simulink model "mrefrobotarm_modified_previous_y_previous_u_previous_ref"  (R2018b)
settings: Solver=FixedStepAuto  StartTime=0.0  StopTime=10  RelTol=1e-3  AbsTol=1e-6
undefined symbols (not defined in the file or in its folder): options, sfunxy2
libraries: neural x949, simulink x1
(part 7 of 31)

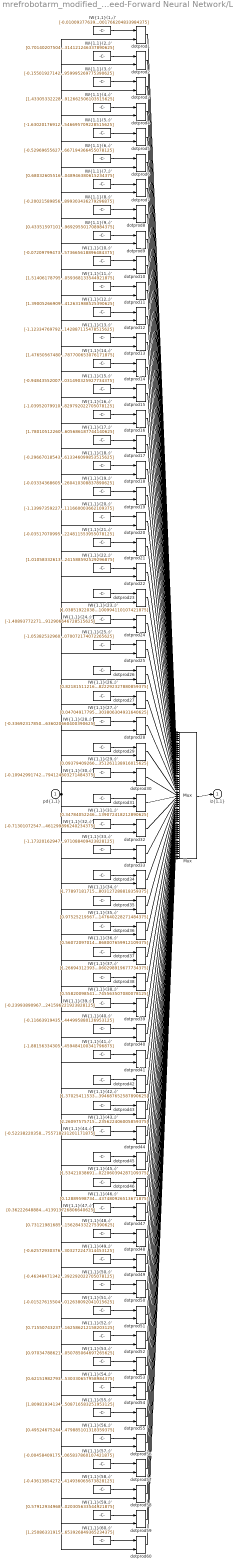
== system mrefrobotarm_modified_previous_y_previous_u_previous_ref/Feed-Forward Neural Network/Layer 1/IW{1,1} ==
  "pd{1,1}" : Inport  PortDimensions=8
      mask Display: e = 0.06;c1 = [120 230 180]/255;c2 = ([120 230 180]+0)/(256+128);c3 = ([120 230 180]+128)/(256+128);patch([0 1 1 0],[0 0 1 1],c1);patch([0 1 1 1-e 1-e 0+e],[0 0 1 1-e 0+e 0+e],c2);patch([0 0 1 1-e 0+e 0+e],[0 1 1 1-e 1-e 0+e],c3);plot([0 1 1 0 0],[0 0 1 1 0]);
  "IW{1,1}(1,:)'" : Constant  Value=[-0.01009377639347205403430596248881556675769388675689697265625;-0.81917856322471305219323767232708632946014404296875;-1.0919884952677578748847508904873393476009368896484375;-0.3232934690770914443191941245459020137786865234375;1.0371983069879358030362936915480531752109527587890625;0.332566501638959455267041676052031107246875762939453125;-0.72214891052584950781323414048529230058193206787109375;0.41554839927694986467798798912554048001766204833984375]
      mask Display: e = 0.06;c1 = [120 150 230]/255;c2 = ([120 150 230]+0)/383;c3 = ([120 150 230]+128)/383;patch([0 1 1 0],[0 0 1 1],c1);patch([0 1 1 1-e 1-e 0+e],[0 0 1 1-e 0+e 0+e],c2);patch([0 0 1 1-e 0+e 0+e],[0 1 1 1-e 1-e 0+e],c3);plot([0 1 1 0 0],[0 0 1 1 0]);disp('Weights');
  "IW{1,1}(10,:)'" : Constant  Value=[-0.0720979947310176616515065006751683540642261505126953125;1.1315755262161395489073356657172553241252899169921875;-0.69309946443650216618692638803622685372829437255859375;-0.1580631105350375487095249127378338016569614410400390625;-0.70708492198913841519924972089938819408416748046875;-0.9763414859311836391242422905634157359600067138671875;0.56334312317556867188983460437157191336154937744140625;-0.319187622528195491522495785829960368573665618896484375]
      mask Display: e = 0.06;c1 = [120 150 230]/255;c2 = ([120 150 230]+0)/383;c3 = ([120 150 230]+128)/383;patch([0 1 1 0],[0 0 1 1],c1);patch([0 1 1 1-e 1-e 0+e],[0 0 1 1-e 0+e 0+e],c2);patch([0 0 1 1-e 0+e 0+e],[0 1 1 1-e 1-e 0+e],c3);plot([0 1 1 0 0],[0 0 1 1 0]);disp('Weights');
  "IW{1,1}(11,:)'" : Constant  Value=[1.514061787956713533986885522608645260334014892578125;-0.41268670620541703097927666021860204637050628662109375;-0.133355521691774558945553508237935602664947509765625;1.4642596982166242725043048267252743244171142578125;-0.92497175926368180309822264462127350270748138427734375;-0.0687966183859873847694643700378946959972381591796875;0.715766413497218589867543414584361016750335693359375;0.2974930277251821575390522411908023059368133544921875]
      mask Display: e = 0.06;c1 = [120 150 230]/255;c2 = ([120 150 230]+0)/383;c3 = ([120 150 230]+128)/383;patch([0 1 1 0],[0 0 1 1],c1);patch([0 1 1 1-e 1-e 0+e],[0 0 1 1-e 0+e 0+e],c2);patch([0 0 1 1-e 0+e 0+e],[0 1 1 1-e 1-e 0+e],c3);plot([0 1 1 0 0],[0 0 1 1 0]);disp('Weights');
  "IW{1,1}(12,:)'" : Constant  Value=[1.390052669090437120757997035980224609375;0.002873883030498494174642676313169431523419916629791259765625;-0.265197877421132155451033440840546973049640655517578125;-0.2012360557710944630738225669119856320321559906005859375;-0.73320460680185417512433332376531325280666351318359375;-0.0226500905621143909518533376967752701602876186370849609375;-0.057008062463787374796186924186258693225681781768798828125;-0.9276377305383221028023399412631988525390625]
      mask Display: e = 0.06;c1 = [120 150 230]/255;c2 = ([120 150 230]+0)/383;c3 = ([120 150 230]+128)/383;patch([0 1 1 0],[0 0 1 1],c1);patch([0 1 1 1-e 1-e 0+e],[0 0 1 1-e 0+e 0+e],c2);patch([0 0 1 1-e 0+e 0+e],[0 1 1 1-e 1-e 0+e],c3);plot([0 1 1 0 0],[0 0 1 1 0]);disp('Weights');
  "IW{1,1}(13,:)'" : Constant  Value=[-1.1233476979256022953990168389282189309597015380859375;-1.2393693114673052235730210668407380580902099609375;0.7914246902064994149128551725880242884159088134765625;-0.274134462483511198716001899811089970171451568603515625;-0.7315570973101059859544648134033195674419403076171875;0.428567667581298328283168075358844362199306488037109375;1.018170137932393526369878600235097110271453857421875;0.49897495766321908750029479051590897142887115478515625]
      mask Display: e = 0.06;c1 = [120 150 230]/255;c2 = ([120 150 230]+0)/383;c3 = ([120 150 230]+128)/383;patch([0 1 1 0],[0 0 1 1],c1);patch([0 1 1 1-e 1-e 0+e],[0 0 1 1-e 0+e 0+e],c2);patch([0 0 1 1-e 0+e 0+e],[0 1 1 1-e 1-e 0+e],c3);plot([0 1 1 0 0],[0 0 1 1 0]);disp('Weights');
  "IW{1,1}(14,:)'" : Constant  Value=[1.4765056748086795579411045764572918415069580078125;-0.90659967261472174104852683740318752825260162353515625;1.1508044721540480193056055213673971593379974365234375;-1.0136176640992273778607568601728416979312896728515625;-0.07767755483619455392219066425241180695593357086181640625;0.57299887905671254006989556728512980043888092041015625;0.449131233253424244633578155116993002593517303466796875;0.1613292379590309522097157923781196586787700653076171875]
      mask Display: e = 0.06;c1 = [120 150 230]/255;c2 = ([120 150 230]+0)/383;c3 = ([120 150 230]+128)/383;patch([0 1 1 0],[0 0 1 1],c1);patch([0 1 1 1-e 1-e 0+e],[0 0 1 1-e 0+e 0+e],c2);patch([0 0 1 1-e 0+e 0+e],[0 1 1 1-e 1-e 0+e],c3);plot([0 1 1 0 0],[0 0 1 1 0]);disp('Weights');
  "IW{1,1}(15,:)'" : Constant  Value=[-0.94843552007180209617587252068915404379367828369140625;-0.455396495188023886502293180456035770475864410400390625;-0.71794256963177804919951086048968136310577392578125;-0.259356227336552891404863885327358730137348175048828125;-0.6977913420825629930988043270190246403217315673828125;1.4367856825259675002115500319632701575756072998046875;0.38097748667274744516220152945606969296932220458984375;-1.2386509874698869992926120175980031490325927734375]
      mask Display: e = 0.06;c1 = [120 150 230]/255;c2 = ([120 150 230]+0)/383;c3 = ([120 150 230]+128)/383;patch([0 1 1 0],[0 0 1 1],c1);patch([0 1 1 1-e 1-e 0+e],[0 0 1 1-e 0+e 0+e],c2);patch([0 0 1 1-e 0+e 0+e],[0 1 1 1-e 1-e 0+e],c3);plot([0 1 1 0 0],[0 0 1 1 0]);disp('Weights');
  "IW{1,1}(16,:)'" : Constant  Value=[-1.03952079910626782321969585609622299671173095703125;0.274781364075693590454108061749138869345188140869140625;-1.0171273753363585523601386739755980670452117919921875;-0.03878824548100874569644958000935730524361133575439453125;0.193393524233432978487456921357079409062862396240234375;0.832640986442755082208577732671983540058135986328125;-0.7503621573611758410748961978242732584476470947265625;-1.01693222204544486686472737346775829792022705078125]
      mask Display: e = 0.06;c1 = [120 150 230]/255;c2 = ([120 150 230]+0)/383;c3 = ([120 150 230]+128)/383;patch([0 1 1 0],[0 0 1 1],c1);patch([0 1 1 1-e 1-e 0+e],[0 0 1 1-e 0+e 0+e],c2);patch([0 0 1 1-e 0+e 0+e],[0 1 1 1-e 1-e 0+e],c3);plot([0 1 1 0 0],[0 0 1 1 0]);disp('Weights');
  "IW{1,1}(17,:)'" : Constant  Value=[1.7801051226057931220481123091303743422031402587890625;1.3780535999959975246298427009605802595615386962890625;0.1885363073008298473443034026786335743963718414306640625;0.365832667926227206312006501320865936577320098876953125;0.6397823368767736607054530395544134080410003662109375;0.379418365358508646867363722776644863188266754150390625;-0.26533033038375464229829958640038967132568359375;0.30752361343576029018009876381256617605686187744140625]
      mask Display: e = 0.06;c1 = [120 150 230]/255;c2 = ([120 150 230]+0)/383;c3 = ([120 150 230]+128)/383;patch([0 1 1 0],[0 0 1 1],c1);patch([0 1 1 1-e 1-e 0+e],[0 0 1 1-e 0+e 0+e],c2);patch([0 0 1 1-e 0+e 0+e],[0 1 1 1-e 1-e 0+e],c3);plot([0 1 1 0 0],[0 0 1 1 0]);disp('Weights');
  "IW{1,1}(18,:)'" : Constant  Value=[-0.296670185432604427422376147660543210804462432861328125;-0.376072809350395387273380265469313599169254302978515625;-0.742727493493180901396044646389782428741455078125;0.86593116784423240783752362403902225196361541748046875;1.37064929615764707904190800036303699016571044921875;-0.59077170502804399188079287341679446399211883544921875;-0.150853642388064368429212436240050010383129119873046875;-0.81451885680998670213881496238172985613346099853515625]
      mask Display: e = 0.06;c1 = [120 150 230]/255;c2 = ([120 150 230]+0)/383;c3 = ([120 150 230]+128)/383;patch([0 1 1 0],[0 0 1 1],c1);patch([0 1 1 1-e 1-e 0+e],[0 0 1 1-e 0+e 0+e],c2);patch([0 0 1 1-e 0+e 0+e],[0 1 1 1-e 1-e 0+e],c3);plot([0 1 1 0 0],[0 0 1 1 0]);disp('Weights');
  "IW{1,1}(19,:)'" : Constant  Value=[-0.033343686056520986660256511413535918109118938446044921875;-0.5300304829595254840768348003621213138103485107421875;-0.66380007316216460555580169966560788452625274658203125;1.4047136071211827612614797544665634632110595703125;-1.4498046029545166302199277197360061109066009521484375;0.60291678893256517302035035754670388996601104736328125;-0.08866355731311535703920156947788200341165065765380859375;-0.3794826026320132772440274493419565260410308837890625]
      mask Display: e = 0.06;c1 = [120 150 230]/255;c2 = ([120 150 230]+0)/383;c3 = ([120 150 230]+128)/383;patch([0 1 1 0],[0 0 1 1],c1);patch([0 1 1 1-e 1-e 0+e],[0 0 1 1-e 0+e 0+e],c2);patch([0 0 1 1-e 0+e 0+e],[0 1 1 1-e 1-e 0+e],c3);plot([0 1 1 0 0],[0 0 1 1 0]);disp('Weights');
  "IW{1,1}(2,:)'" : Constant  Value=[0.70140207504615859068763938921620137989521026611328125;0.50190548995443251545367502330918796360492706298828125;1.178018179952304844704258357523940503597259521484375;1.2397835887663470888497840860509313642978668212890625;1.2796434023332323715038683076272718608379364013671875;-0.91185964599935942498376562070916406810283660888671875;-0.53150803539821700471890153494314290583133697509765625;0.60564464089634706400744335041963495314121246337890625]
      mask Display: e = 0.06;c1 = [120 150 230]/255;c2 = ([120 150 230]+0)/383;c3 = ([120 150 230]+128)/383;patch([0 1 1 0],[0 0 1 1],c1);patch([0 1 1 1-e 1-e 0+e],[0 0 1 1-e 0+e 0+e],c2);patch([0 0 1 1-e 0+e 0+e],[0 1 1 1-e 1-e 0+e],c3);plot([0 1 1 0 0],[0 0 1 1 0]);disp('Weights');
  "IW{1,1}(20,:)'" : Constant  Value=[-1.139973592271053437485761605785228312015533447265625;0.922414963173714408384284979547373950481414794921875;0.573062580631909401773782519740052521228790283203125;-1.0638984585657997872232272129622288048267364501953125;0.26000003990170894585531868870020844042301177978515625;-1.0082968466580883859506911903736181557178497314453125;-0.427975846736409037962545198752195574343204498291015625;-0.404524086197522725338870941413915716111660003662109375]
      mask Display: e = 0.06;c1 = [120 150 230]/255;c2 = ([120 150 230]+0)/383;c3 = ([120 150 230]+128)/383;patch([0 1 1 0],[0 0 1 1],c1);patch([0 1 1 1-e 1-e 0+e],[0 0 1 1-e 0+e 0+e],c2);patch([0 0 1 1-e 0+e 0+e],[0 1 1 1-e 1-e 0+e],c3);plot([0 1 1 0 0],[0 0 1 1 0]);disp('Weights');
  "IW{1,1}(21,:)'" : Constant  Value=[-0.035170709953433833272473663100754492916166782379150390625;-0.2048825226713566205472005776755395345389842987060546875;1.02054460527438362049679199117235839366912841796875;-1.0483393952073327692886550721595995128154754638671875;0.218116613354659649726130510316579602658748626708984375;-1.2810290950311611357648189368774183094501495361328125;0.9860421910966181702207222770084626972675323486328125;-0.30606358720429505115845358886872418224811553955078125]
      mask Display: e = 0.06;c1 = [120 150 230]/255;c2 = ([120 150 230]+0)/383;c3 = ([120 150 230]+128)/383;patch([0 1 1 0],[0 0 1 1],c1);patch([0 1 1 1-e 1-e 0+e],[0 0 1 1-e 0+e 0+e],c2);patch([0 0 1 1-e 0+e 0+e],[0 1 1 1-e 1-e 0+e],c3);plot([0 1 1 0 0],[0 0 1 1 0]);disp('Weights');
  "IW{1,1}(22,:)'" : Constant  Value=[1.010583326137901583052780551952309906482696533203125;-0.34255096084721647908821751116192899644374847412109375;0.49744289643764882935528248708578757941722869873046875;0.81639407608297276386366547740180976688861846923828125;0.268321118702407546141586180965532548725605010986328125;-1.0453340103508159675271826927200891077518463134765625;1.0355195133497721027282523209578357636928558349609375;-0.53749069554478612342762744447099976241588592529296875]
      mask Display: e = 0.06;c1 = [120 150 230]/255;c2 = ([120 150 230]+0)/383;c3 = ([120 150 230]+128)/383;patch([0 1 1 0],[0 0 1 1],c1);patch([0 1 1 1-e 1-e 0+e],[0 0 1 1-e 0+e 0+e],c2);patch([0 0 1 1-e 0+e 0+e],[0 1 1 1-e 1-e 0+e],c3);plot([0 1 1 0 0],[0 0 1 1 0]);disp('Weights');
  "IW{1,1}(23,:)'" : Constant  Value=[1.038519220380671459480481644277460873126983642578125;0.833366743499137196948822747799567878246307373046875;1.2577080160119058493961574640707112848758697509765625;-0.401936187267794731159398224917822517454624176025390625;0.04902228607691017092662377763190306723117828369140625;-0.54247854896119485079708510966156609356403350830078125;-1.039179720087923808335972353233955800533294677734375;-0.5448646607404519226491856898064725100994110107421875]
      mask Display: e = 0.06;c1 = [120 150 230]/255;c2 = ([120 150 230]+0)/383;c3 = ([120 150 230]+128)/383;patch([0 1 1 0],[0 0 1 1],c1);patch([0 1 1 1-e 1-e 0+e],[0 0 1 1-e 0+e 0+e],c2);patch([0 0 1 1-e 0+e 0+e],[0 1 1 1-e 1-e 0+e],c3);plot([0 1 1 0 0],[0 0 1 1 0]);disp('Weights');
  "IW{1,1}(24,:)'" : Constant  Value=[-1.4089377227153281335603196566808037459850311279296875;0.77299854810514367908780286597902886569499969482421875;0.309547994905805035070756048298790119588375091552734375;-0.279630711329400372111564365695812739431858062744140625;-1.453337035422787248961640216293744742870330810546875;0.139437025698908978466050712086143903434276580810546875;-0.56209102683994849325443965426529757678508758544921875;0.59696878013546650354470557431341148912906646728515625]
      mask Display: e = 0.06;c1 = [120 150 230]/255;c2 = ([120 150 230]+0)/383;c3 = ([120 150 230]+128)/383;patch([0 1 1 0],[0 0 1 1],c1);patch([0 1 1 1-e 1-e 0+e],[0 0 1 1-e 0+e 0+e],c2);patch([0 0 1 1-e 0+e 0+e],[0 1 1 1-e 1-e 0+e],c3);plot([0 1 1 0 0],[0 0 1 1 0]);disp('Weights');
  "IW{1,1}(25,:)'" : Constant  Value=[-1.053825329600287741271813501953147351741790771484375;2.104248436455582460524738053209148347377777099609375;-1.389722016511392599369401068543083965778350830078125;0.70194513487137377705238350245053879916667938232421875;0.016033632287981595954118319014014559797942638397216796875;0.726493334124701295451131954905577003955841064453125;-0.138938571659139586955689082969911396503448486328125;0.48164231672507418213768914938555099070072174072265625]
      mask Display: e = 0.06;c1 = [120 150 230]/255;c2 = ([120 150 230]+0)/383;c3 = ([120 150 230]+128)/383;patch([0 1 1 0],[0 0 1 1],c1);patch([0 1 1 1-e 1-e 0+e],[0 0 1 1-e 0+e 0+e],c2);patch([0 0 1 1-e 0+e 0+e],[0 1 1 1-e 1-e 0+e],c3);plot([0 1 1 0 0],[0 0 1 1 0]);disp('Weights');
  "IW{1,1}(26,:)'" : Constant  Value=[0.8218151121617001120256418289500288665294647216796875;1.237877827933333119148073819815181195735931396484375;0.578162601622759897423975417041219770908355712890625;-0.90524346095929486555320409024716354906558990478515625;-0.557227828939628633264646850875578820705413818359375;0.693063774200946891568264618399553000926971435546875;0.848423865073127725366930462769232690334320068359375;-0.7998183010585433461159254875383339822292327880859375]
      mask Display: e = 0.06;c1 = [120 150 230]/255;c2 = ([120 150 230]+0)/383;c3 = ([120 150 230]+128)/383;patch([0 1 1 0],[0 0 1 1],c1);patch([0 1 1 1-e 1-e 0+e],[0 0 1 1-e 0+e 0+e],c2);patch([0 0 1 1-e 0+e 0+e],[0 1 1 1-e 1-e 0+e],c3);plot([0 1 1 0 0],[0 0 1 1 0]);disp('Weights');
  "IW{1,1}(27,:)'" : Constant  Value=[0.047049177951239286310514131628224276937544345855712890625;-0.491975786566918704689754804348922334611415863037109375;1.2519795722981628127712383502512238919734954833984375;-0.54908256817673317673467181521118618547916412353515625;-0.65890045944206165895451476899324916303157806396484375;-0.2162576647712697586189989351623808033764362335205078125;-0.09278042821038166854119566551162279210984706878662109375;0.472893608075191596018527206979342736303806304931640625]
      mask Display: e = 0.06;c1 = [120 150 230]/255;c2 = ([120 150 230]+0)/383;c3 = ([120 150 230]+128)/383;patch([0 1 1 0],[0 0 1 1],c1);patch([0 1 1 1-e 1-e 0+e],[0 0 1 1-e 0+e 0+e],c2);patch([0 0 1 1-e 0+e 0+e],[0 1 1 1-e 1-e 0+e],c3);plot([0 1 1 0 0],[0 0 1 1 0]);disp('Weights');
  "IW{1,1}(28,:)'" : Constant  Value=[-0.3369231785042738902546943791094236075878143310546875;-0.181984775034675860805322145097306929528713226318359375;0.72097050985835930969614082641783170402050018310546875;0.389238215915795715549307942637824453413486480712890625;1.1885279226217166925749779693433083593845367431640625;-0.2162301922323874026066192755024530924856662750244140625;-0.55743284950293936486076518121990375220775604248046875;1.0239338395360386702037658324115909636020660400390625]
      mask Display: e = 0.06;c1 = [120 150 230]/255;c2 = ([120 150 230]+0)/383;c3 = ([120 150 230]+128)/383;patch([0 1 1 0],[0 0 1 1],c1);patch([0 1 1 1-e 1-e 0+e],[0 0 1 1-e 0+e 0+e],c2);patch([0 0 1 1-e 0+e 0+e],[0 1 1 1-e 1-e 0+e],c3);plot([0 1 1 0 0],[0 0 1 1 0]);disp('Weights');
  "IW{1,1}(29,:)'" : Constant  Value=[0.09379409266803222233743753122325870208442211151123046875;0.8258233160961461205573641564114950597286224365234375;1.3081801207924230734391812802641652524471282958984375;0.1938697051900289125558884961719741113483905792236328125;0.573395538471701993188389678834937512874603271484375;-0.7356971128263525283585977376787923276424407958984375;0.182430235492571923838767133929650299251079559326171875;-1.25940850979900265116384616703726351261138916015625]
      mask Display: e = 0.06;c1 = [120 150 230]/255;c2 = ([120 150 230]+0)/383;c3 = ([120 150 230]+128)/383;patch([0 1 1 0],[0 0 1 1],c1);patch([0 1 1 1-e 1-e 0+e],[0 0 1 1-e 0+e 0+e],c2);patch([0 0 1 1-e 0+e 0+e],[0 1 1 1-e 1-e 0+e],c3);plot([0 1 1 0 0],[0 0 1 1 0]);disp('Weights');
  "IW{1,1}(3,:)'" : Constant  Value=[-0.1550192714260813786619763732232968322932720184326171875;0.267682004821501784430637371769989840686321258544921875;0.8213433311036910655644760481663979589939117431640625;0.2482384568506261768305876103113405406475067138671875;-0.61724220880742508565930393160670064389705657958984375;-0.79902255865863003325699764900491572916507720947265625;1.29132611134465502544799164752475917339324951171875;0.7532613633114204620966347647481597959995269775390625]
      mask Display: e = 0.06;c1 = [120 150 230]/255;c2 = ([120 150 230]+0)/383;c3 = ([120 150 230]+128)/383;patch([0 1 1 0],[0 0 1 1],c1);patch([0 1 1 1-e 1-e 0+e],[0 0 1 1-e 0+e 0+e],c2);patch([0 0 1 1-e 0+e 0+e],[0 1 1 1-e 1-e 0+e],c3);plot([0 1 1 0 0],[0 0 1 1 0]);disp('Weights');
  "IW{1,1}(30,:)'" : Constant  Value=[-0.10942991742337003502338887983569293282926082611083984375;-0.96617865662847624008691127528436481952667236328125;1.22815391380386440545180448680184781551361083984375;0.9209715069928978703472921552020125091075897216796875;-0.87794222936966936909897185614681802690029144287109375;0.58692975040539197006950189461349509656429290771484375;0.03017362296723884174109997502455371432006359100341796875;-0.90446550378048884422099717994569800794124603271484375]
      mask Display: e = 0.06;c1 = [120 150 230]/255;c2 = ([120 150 230]+0)/383;c3 = ([120 150 230]+128)/383;patch([0 1 1 0],[0 0 1 1],c1);patch([0 1 1 1-e 1-e 0+e],[0 0 1 1-e 0+e 0+e],c2);patch([0 0 1 1-e 0+e 0+e],[0 1 1 1-e 1-e 0+e],c3);plot([0 1 1 0 0],[0 0 1 1 0]);disp('Weights');
  "IW{1,1}(31,:)'" : Constant  Value=[0.34784052246623431425831540764193050563335418701171875;0.7424319382244732867803804765571840107440948486328125;0.89792498586287472495115480342064984142780303955078125;1.099066964391795409028418362140655517578125;0.00058579181141991433501292618757361196912825107574462890625;-0.89695655979727340056939510759548284113407135009765625;1.25394388993594230186090499046258628368377685546875;0.90635322106720261903234359124326147139072418212890625]
      mask Display: e = 0.06;c1 = [120 150 230]/255;c2 = ([120 150 230]+0)/383;c3 = ([120 150 230]+128)/383;patch([0 1 1 0],[0 0 1 1],c1);patch([0 1 1 1-e 1-e 0+e],[0 0 1 1-e 0+e 0+e],c2);patch([0 0 1 1-e 0+e 0+e],[0 1 1 1-e 1-e 0+e],c3);plot([0 1 1 0 0],[0 0 1 1 0]);disp('Weights');
  "IW{1,1}(32,:)'" : Constant  Value=[-0.71301072547602017959178510864148847758769989013671875;0.5241561595862809230794709947076626121997833251953125;0.3885115679967781066039833604008890688419342041015625;-0.69944953560710987350290679387398995459079742431640625;1.2447082577953547666282929640146903693675994873046875;0.3781402687772514870090390104451216757297515869140625;-1.0318004731634136117435218693572096526622772216796875;0.936380669930056086514014168642461299896240234375]
      mask Display: e = 0.06;c1 = [120 150 230]/255;c2 = ([120 150 230]+0)/383;c3 = ([120 150 230]+128)/383;patch([0 1 1 0],[0 0 1 1],c1);patch([0 1 1 1-e 1-e 0+e],[0 0 1 1-e 0+e 0+e],c2);patch([0 0 1 1-e 0+e 0+e],[0 1 1 1-e 1-e 0+e],c3);plot([0 1 1 0 0],[0 0 1 1 0]);disp('Weights');
  "IW{1,1}(33,:)'" : Constant  Value=[-1.1732016294754872287597891045152209699153900146484375;-0.422969128171088615264494592338451184332370758056640625;0.54255586269967881474229898230987600982189178466796875;-0.73308841281237679954330133114126510918140411376953125;-0.97167834539178798980429974108119495213031768798828125;-1.202198002474001103934142520301975309848785400390625;-0.348202785759618882455157518052146770060062408447265625;-1.205837459930009902819847411592490971088409423828125]
      mask Display: e = 0.06;c1 = [120 150 230]/255;c2 = ([120 150 230]+0)/383;c3 = ([120 150 230]+128)/383;patch([0 1 1 0],[0 0 1 1],c1);patch([0 1 1 1-e 1-e 0+e],[0 0 1 1-e 0+e 0+e],c2);patch([0 0 1 1-e 0+e 0+e],[0 1 1 1-e 1-e 0+e],c3);plot([0 1 1 0 0],[0 0 1 1 0]);disp('Weights');
  "IW{1,1}(34,:)'" : Constant  Value=[1.77897181715445906746708715218119323253631591796875;-0.280453940129275436365929863313795067369937896728515625;0.367343171050295402846330716783995740115642547607421875;-1.008703116569453772655151624348945915699005126953125;0.2803758972512444547220411550370045006275177001953125;0.74306829139624663849161834150436334311962127685546875;-0.279494497759325277730368952688877470791339874267578125;0.98768799744963187148272254489711485803127288818359375]
      mask Display: e = 0.06;c1 = [120 150 230]/255;c2 = ([120 150 230]+0)/383;c3 = ([120 150 230]+128)/383;patch([0 1 1 0],[0 0 1 1],c1);patch([0 1 1 1-e 1-e 0+e],[0 0 1 1-e 0+e 0+e],c2);patch([0 0 1 1-e 0+e 0+e],[0 1 1 1-e 1-e 0+e],c3);plot([0 1 1 0 0],[0 0 1 1 0]);disp('Weights');
  "IW{1,1}(35,:)'" : Constant  Value=[0.97525219567861320957291582089965231716632843017578125;0.88646219952508398254309440744691528379917144775390625;-1.730996619538126335413608103408478200435638427734375;0.0396632946371748007496904619983979500830173492431640625;-0.409742039261921764392582190339453518390655517578125;-0.3665493088119438080951795200235210359096527099609375;1.41189287226400050911934158648364245891571044921875;0.0695407452994048769223667250116704963147640228271484375]
      mask Display: e = 0.06;c1 = [120 150 230]/255;c2 = ([120 150 230]+0)/383;c3 = ([120 150 230]+128)/383;patch([0 1 1 0],[0 0 1 1],c1);patch([0 1 1 1-e 1-e 0+e],[0 0 1 1-e 0+e 0+e],c2);patch([0 0 1 1-e 0+e 0+e],[0 1 1 1-e 1-e 0+e],c3);plot([0 1 1 0 0],[0 0 1 1 0]);disp('Weights');
  "IW{1,1}(36,:)'" : Constant  Value=[0.56072097014748345511492289006127975881099700927734375;-0.469901980631740989746703007767791859805583953857421875;0.6628153017091324983312006224878132343292236328125;0.7677647851080724450412162696011364459991455078125;-1.5570532384978843509770740638487040996551513671875;0.55547680871442739469756588732707314193248748779296875;0.399763330482430456758180525866919197142124176025390625;-0.60140820677555628659405329017317853868007659912109375]
      mask Display: e = 0.06;c1 = [120 150 230]/255;c2 = ([120 150 230]+0)/383;c3 = ([120 150 230]+128)/383;patch([0 1 1 0],[0 0 1 1],c1);patch([0 1 1 1-e 1-e 0+e],[0 0 1 1-e 0+e 0+e],c2);patch([0 0 1 1-e 0+e 0+e],[0 1 1 1-e 1-e 0+e],c3);plot([0 1 1 0 0],[0 0 1 1 0]);disp('Weights');
  "IW{1,1}(37,:)'" : Constant  Value=[1.2669431239388433407810907738166861236095428466796875;0.84499757606978864732383271984872408211231231689453125;-0.6865178873488713140460504291695542633533477783203125;0.86809844202686192726758918070117942988872528076171875;0.8608914789270685208322220205445773899555206298828125;1.177957103666323224189227403257973492145538330078125;-0.0379420015788152209523786950740031898021697998046875;-1.075985690857061083391954525723122060298919677734375]
      mask Display: e = 0.06;c1 = [120 150 230]/255;c2 = ([120 150 230]+0)/383;c3 = ([120 150 230]+128)/383;patch([0 1 1 0],[0 0 1 1],c1);patch([0 1 1 1-e 1-e 0+e],[0 0 1 1-e 0+e 0+e],c2);patch([0 0 1 1-e 0+e 0+e],[0 1 1 1-e 1-e 0+e],c3);plot([0 1 1 0 0],[0 0 1 1 0]);disp('Weights');
  "IW{1,1}(38,:)'" : Constant  Value=[0.55820098541315044116117860539816319942474365234375;0.79054831004162406937751939040026627480983734130859375;-0.8874852575703595647382826427929103374481201171875;-1.09062952986268868471597670577466487884521484375;-0.45622805513097752783124860798125155270099639892578125;-0.37040001200239436318639718592748977243900299072265625;-1.189528150446891974212348941364325582981109619140625;-1.116516071350041716669920788262970745563507080078125]
      mask Display: e = 0.06;c1 = [120 150 230]/255;c2 = ([120 150 230]+0)/383;c3 = ([120 150 230]+128)/383;patch([0 1 1 0],[0 0 1 1],c1);patch([0 1 1 1-e 1-e 0+e],[0 0 1 1-e 0+e 0+e],c2);patch([0 0 1 1-e 0+e 0+e],[0 1 1 1-e 1-e 0+e],c3);plot([0 1 1 0 0],[0 0 1 1 0]);disp('Weights');
  "IW{1,1}(39,:)'" : Constant  Value=[-0.2399389096781732455543334481262718327343463897705078125;1.3447224058359446008381610226933844387531280517578125;-1.38142976173474618661884960602037608623504638671875;0.474640863170868343434705138861318118870258331298828125;-0.1470266327579221321553148982275160960853099822998046875;-0.67018418152759551276176352985203266143798828125;-0.59239089958121649015510001845541410148143768310546875;0.1371346520832968096659243428803165443241596221923828125]
      mask Display: e = 0.06;c1 = [120 150 230]/255;c2 = ([120 150 230]+0)/383;c3 = ([120 150 230]+128)/383;patch([0 1 1 0],[0 0 1 1],c1);patch([0 1 1 1-e 1-e 0+e],[0 0 1 1-e 0+e 0+e],c2);patch([0 0 1 1-e 0+e 0+e],[0 1 1 1-e 1-e 0+e],c3);plot([0 1 1 0 0],[0 0 1 1 0]);disp('Weights');
  "IW{1,1}(4,:)'" : Constant  Value=[1.4330533222863213183018160634674131870269775390625;-0.09029904425561195713267892415387905202805995941162109375;-0.1378620578092981940887540304174763150513172149658203125;-0.128678062876721510665589676136733032763004302978515625;0.700090148025589886771058445447124540805816650390625;0.59531505529047235025785766993067227303981781005859375;-0.08226765583024404915324367948414874263107776641845703125;1.066435135058397154494969072402454912662506103515625]
      mask Display: e = 0.06;c1 = [120 150 230]/255;c2 = ([120 150 230]+0)/383;c3 = ([120 150 230]+128)/383;patch([0 1 1 0],[0 0 1 1],c1);patch([0 1 1 1-e 1-e 0+e],[0 0 1 1-e 0+e 0+e],c2);patch([0 0 1 1-e 0+e 0+e],[0 1 1 1-e 1-e 0+e],c3);plot([0 1 1 0 0],[0 0 1 1 0]);disp('Weights');
  "IW{1,1}(40,:)'" : Constant  Value=[-0.1166391943536552455729093935588025487959384918212890625;1.3594486796418383534046370186842978000640869140625;0.57698100738084712180153701410745270550251007080078125;-0.059919148073443929958248332923176349140703678131103515625;-0.789043368311738380072029030998237431049346923828125;-0.86628954342663500032273304896079935133457183837890625;0.14402892035788161795295536649064160883426666259765625;-0.913235673254125135400727231171913444995880126953125]
      mask Display: e = 0.06;c1 = [120 150 230]/255;c2 = ([120 150 230]+0)/383;c3 = ([120 150 230]+128)/383;patch([0 1 1 0],[0 0 1 1],c1);patch([0 1 1 1-e 1-e 0+e],[0 0 1 1-e 0+e 0+e],c2);patch([0 0 1 1-e 0+e 0+e],[0 1 1 1-e 1-e 0+e],c3);plot([0 1 1 0 0],[0 0 1 1 0]);disp('Weights');
  "IW{1,1}(41,:)'" : Constant  Value=[-1.881563343058816339947725282399915158748626708984375;0.9950257472784775902852061335579492151737213134765625;0.93709934505314451680391130139469169080257415771484375;-0.7473708296793655225798147512250579893589019775390625;-0.454191669232585137905289229820482432842254638671875;0.31070247408903550745407073918613605201244354248046875;-0.177938424903270664412247015206958167254924774169921875;-0.9237690427451343833098462710040621459484100341796875]
      mask Display: e = 0.06;c1 = [120 150 230]/255;c2 = ([120 150 230]+0)/383;c3 = ([120 150 230]+128)/383;patch([0 1 1 0],[0 0 1 1],c1);patch([0 1 1 1-e 1-e 0+e],[0 0 1 1-e 0+e 0+e],c2);patch([0 0 1 1-e 0+e 0+e],[0 1 1 1-e 1-e 0+e],c3);plot([0 1 1 0 0],[0 0 1 1 0]);disp('Weights');
  "IW{1,1}(42,:)'" : Constant  Value=[1.3702541153334115708872786854044534265995025634765625;-0.1156131328774818722848749530385248363018035888671875;0.614274810825514716583484187140129506587982177734375;0.318766942419542453901470935306861065328121185302734375;1.2991946873100921333588075867737643420696258544921875;-0.5215118465581591866708777160965837538242340087890625;0.565289984710197312978152694995515048503875732421875;0.9677004451813824292827348472201265394687652587890625]
      mask Display: e = 0.06;c1 = [120 150 230]/255;c2 = ([120 150 230]+0)/383;c3 = ([120 150 230]+128)/383;patch([0 1 1 0],[0 0 1 1],c1);patch([0 1 1 1-e 1-e 0+e],[0 0 1 1-e 0+e 0+e],c2);patch([0 0 1 1-e 0+e 0+e],[0 1 1 1-e 1-e 0+e],c3);plot([0 1 1 0 0],[0 0 1 1 0]);disp('Weights');
  "IW{1,1}(43,:)'" : Constant  Value=[2.260975757154053855657593885553069412708282470703125;-2.1510199031089261012539282091893255710601806640625;-0.077576990798844891461527595311054028570652008056640625;-0.4821861293228300038293809848255477845668792724609375;-0.365668656400341240964024791537667624652385711669921875;0.13451908107684185100794138634228147566318511962890625;0.232971221479439716262049842043779790401458740234375;-0.56912634940822426354856133912107907235622406005859375]
      mask Display: e = 0.06;c1 = [120 150 230]/255;c2 = ([120 150 230]+0)/383;c3 = ([120 150 230]+128)/383;patch([0 1 1 0],[0 0 1 1],c1);patch([0 1 1 1-e 1-e 0+e],[0 0 1 1-e 0+e 0+e],c2);patch([0 0 1 1-e 0+e 0+e],[0 1 1 1-e 1-e 0+e],c3);plot([0 1 1 0 0],[0 0 1 1 0]);disp('Weights');
  "IW{1,1}(44,:)'" : Constant  Value=[-0.5223822035888729953256870430777780711650848388671875;-0.419199451858211669108555952334427274763584136962890625;0.312152287994981680885331343233701772987842559814453125;-0.39644961503704989613794396063894964754581451416015625;0.10427136538485380634622146089895977638661861419677734375;0.308491948074407051905154730775393545627593994140625;1.304266392973596477844466789974831044673919677734375;1.1619200009825803032725843877415172755718231201171875]
      mask Display: e = 0.06;c1 = [120 150 230]/255;c2 = ([120 150 230]+0)/383;c3 = ([120 150 230]+128)/383;patch([0 1 1 0],[0 0 1 1],c1);patch([0 1 1 1-e 1-e 0+e],[0 0 1 1-e 0+e 0+e],c2);patch([0 0 1 1-e 0+e 0+e],[0 1 1 1-e 1-e 0+e],c3);plot([0 1 1 0 0],[0 0 1 1 0]);disp('Weights');
  "IW{1,1}(45,:)'" : Constant  Value=[1.534210386911081247518495729309506714344024658203125;-0.36943060246236936183805710243177600204944610595703125;-1.3810021468498721031181730722892098128795623779296875;1.937610501525079076401425481890328228473663330078125;-0.091496085529782889000927070810575969517230987548828125;-1.093079792816382678211084567010402679443359375;1.0732569773862798978569799146498553454875946044921875;-0.401897835916557644164726070812321268022060394287109375]
      mask Display: e = 0.06;c1 = [120 150 230]/255;c2 = ([120 150 230]+0)/383;c3 = ([120 150 230]+128)/383;patch([0 1 1 0],[0 0 1 1],c1);patch([0 1 1 1-e 1-e 0+e],[0 0 1 1-e 0+e 0+e],c2);patch([0 0 1 1-e 0+e 0+e],[0 1 1 1-e 1-e 0+e],c3);plot([0 1 1 0 0],[0 0 1 1 0]);disp('Weights');
  "IW{1,1}(46,:)'" : Constant  Value=[0.1288959873434139813408449981579906307160854339599609375;-0.416959915904302536038272819496341980993747711181640625;0.5385013722251594803225316354655660688877105712890625;0.465201886438678935409285486457520164549350738525390625;-1.7869468184748829031605055206455290317535400390625;0.1867918035887883021484157097802381031215190887451171875;-0.5808952579994126619311600734363310039043426513671875;0.562340466871261934755921174655668437480926513671875]
      mask Display: e = 0.06;c1 = [120 150 230]/255;c2 = ([120 150 230]+0)/383;c3 = ([120 150 230]+128)/383;patch([0 1 1 0],[0 0 1 1],c1);patch([0 1 1 1-e 1-e 0+e],[0 0 1 1-e 0+e 0+e],c2);patch([0 0 1 1-e 0+e 0+e],[0 1 1 1-e 1-e 0+e],c3);plot([0 1 1 0 0],[0 0 1 1 0]);disp('Weights');
  "IW{1,1}(47,:)'" : Constant  Value=[0.36222648884403507718587889030459336936473846435546875;0.5520284332054365972197729206527583301067352294921875;-0.91340259002056656267853895769803784787654876708984375;-0.573216288087723402355777579941786825656890869140625;0.538586801260685366088409864460118114948272705078125;0.990522257548015705452826296095736324787139892578125;0.938203517005444798115831872564740478992462158203125;-0.67821259752334928094796850928105413913726806640625]
      mask Display: e = 0.06;c1 = [120 150 230]/255;c2 = ([120 150 230]+0)/383;c3 = ([120 150 230]+128)/383;patch([0 1 1 0],[0 0 1 1],c1);patch([0 1 1 1-e 1-e 0+e],[0 0 1 1-e 0+e 0+e],c2);patch([0 0 1 1-e 0+e 0+e],[0 1 1 1-e 1-e 0+e],c3);plot([0 1 1 0 0],[0 0 1 1 0]);disp('Weights');
  "IW{1,1}(48,:)'" : Constant  Value=[0.73121981685810177875595172736211679875850677490234375;-0.274634926975565518691979605137021280825138092041015625;0.2147850429710086161971815954530029557645320892333984375;-0.390024797666452760491750950677669607102870941162109375;-1.0355270645634295778592104397830553352832794189453125;-1.2024609516377349205384916785988025367259979248046875;0.57731260016769481158149801558465696871280670166015625;1.091904941611313351046419484191574156284332275390625]
      mask Display: e = 0.06;c1 = [120 150 230]/255;c2 = ([120 150 230]+0)/383;c3 = ([120 150 230]+128)/383;patch([0 1 1 0],[0 0 1 1],c1);patch([0 1 1 1-e 1-e 0+e],[0 0 1 1-e 0+e 0+e],c2);patch([0 0 1 1-e 0+e 0+e],[0 1 1 1-e 1-e 0+e],c3);plot([0 1 1 0 0],[0 0 1 1 0]);disp('Weights');
  "IW{1,1}(49,:)'" : Constant  Value=[-0.62572930376387103645896559100947342813014984130859375;0.192305525516508091232736887832288630306720733642578125;0.29223319201677699918917596733081154525279998779296875;1.10515799470984266150708208442665636539459228515625;1.10419541007198862558880136930383741855621337890625;-0.362041175320139851923073592843138612806797027587890625;0.41853513630726524308300895427237264811992645263671875;-0.93634500517111451944884947806713171303272247314453125]
      mask Display: e = 0.06;c1 = [120 150 230]/255;c2 = ([120 150 230]+0)/383;c3 = ([120 150 230]+128)/383;patch([0 1 1 0],[0 0 1 1],c1);patch([0 1 1 1-e 1-e 0+e],[0 0 1 1-e 0+e 0+e],c2);patch([0 0 1 1-e 0+e 0+e],[0 1 1 1-e 1-e 0+e],c3);plot([0 1 1 0 0],[0 0 1 1 0]);disp('Weights');
  "IW{1,1}(5,:)'" : Constant  Value=[-1.6302017691206389660152353826561011373996734619140625;1.1658952120583834233258357926388271152973175048828125;0.328612534194750782745586548116989433765411376953125;0.057148484511901853633020209599635563790798187255859375;0.10199858774596597121853136513891513459384441375732421875;0.293689141264276809550892721745185554027557373046875;1.3574046633455922883371158604859374463558197021484375;0.52581408090018710854707251201034523546695709228515625]
      mask Display: e = 0.06;c1 = [120 150 230]/255;c2 = ([120 150 230]+0)/383;c3 = ([120 150 230]+128)/383;patch([0 1 1 0],[0 0 1 1],c1);patch([0 1 1 1-e 1-e 0+e],[0 0 1 1-e 0+e 0+e],c2);patch([0 0 1 1-e 0+e 0+e],[0 1 1 1-e 1-e 0+e],c3);plot([0 1 1 0 0],[0 0 1 1 0]);disp('Weights');
  "IW{1,1}(50,:)'" : Constant  Value=[-0.46348471342679520290630534873344004154205322265625;0.144395497249082682689191869940259493887424468994140625;1.569600753927898661999051910242997109889984130859375;0.65189807807301225484053475156542845070362091064453125;1.799031349010675739918951876461505889892578125;0.08719481745500716474150948442911612801253795623779296875;0.38665738953421990853343004346243105828762054443359375;-1.0775093032780482804611210667644627392292022705078125]
      mask Display: e = 0.06;c1 = [120 150 230]/255;c2 = ([120 150 230]+0)/383;c3 = ([120 150 230]+128)/383;patch([0 1 1 0],[0 0 1 1],c1);patch([0 1 1 1-e 1-e 0+e],[0 0 1 1-e 0+e 0+e],c2);patch([0 0 1 1-e 0+e 0+e],[0 1 1 1-e 1-e 0+e],c3);plot([0 1 1 0 0],[0 0 1 1 0]);disp('Weights');
  "IW{1,1}(51,:)'" : Constant  Value=[-0.01527615504234090641755283712655000272206962108612060546875;0.88697721456426370512104995214031077921390533447265625;1.2210882097999109507924231365905143320560455322265625;0.498960703809830319332974113422096706926822662353515625;-1.3793098432327204339031823110417462885379791259765625;-1.1688876275862101206115539753227494657039642333984375;1.325778450150171039467750233598053455352783203125;0.06955829108605073030080490070758969523012638092041015625]
      mask Display: e = 0.06;c1 = [120 150 230]/255;c2 = ([120 150 230]+0)/383;c3 = ([120 150 230]+128)/383;patch([0 1 1 0],[0 0 1 1],c1);patch([0 1 1 1-e 1-e 0+e],[0 0 1 1-e 0+e 0+e],c2);patch([0 0 1 1-e 0+e 0+e],[0 1 1 1-e 1-e 0+e],c3);plot([0 1 1 0 0],[0 0 1 1 0]);disp('Weights');
  "IW{1,1}(52,:)'" : Constant  Value=[0.71550743237089575732312596301198936998844146728515625;-0.865346361151677623269051764509640634059906005859375;1.0974425824873133006320813365164212882518768310546875;0.5965439665360026122442604901152662932872772216796875;-1.010921177194115561093212818377651274204254150390625;-1.0352934979927310710223764544934965670108795166015625;-0.7936580582601122646480007460922934114933013916015625;-0.411364731463568500391403404137236066162586212158203125]
      mask Display: e = 0.06;c1 = [120 150 230]/255;c2 = ([120 150 230]+0)/383;c3 = ([120 150 230]+128)/383;patch([0 1 1 0],[0 0 1 1],c1);patch([0 1 1 1-e 1-e 0+e],[0 0 1 1-e 0+e 0+e],c2);patch([0 0 1 1-e 0+e 0+e],[0 1 1 1-e 1-e 0+e],c3);plot([0 1 1 0 0],[0 0 1 1 0]);disp('Weights');
  "IW{1,1}(53,:)'" : Constant  Value=[0.970347886213300814262083804351277649402618408203125;1.3880928056877552823067389908828772604465484619140625;-0.220359308736878034551409655250608921051025390625;-0.2412131590352391274922894126575556583702564239501953125;-0.56985902808800192875793300117948092520236968994140625;0.40130853779968267414091087630367837846279144287109375;1.2578910474645230710422083575394935905933380126953125;-0.25411460007829111962252000012085773050785064697265625]
      mask Display: e = 0.06;c1 = [120 150 230]/255;c2 = ([120 150 230]+0)/383;c3 = ([120 150 230]+128)/383;patch([0 1 1 0],[0 0 1 1],c1);patch([0 1 1 1-e 1-e 0+e],[0 0 1 1-e 0+e 0+e],c2);patch([0 0 1 1-e 0+e 0+e],[0 1 1 1-e 1-e 0+e],c3);plot([0 1 1 0 0],[0 0 1 1 0]);disp('Weights');
  "IW{1,1}(54,:)'" : Constant  Value=[0.6215198279374003487163236059132032096385955810546875;-1.629635888729266124386185765615664422512054443359375;0.189813216192437350660071615493507124483585357666015625;-0.06836090554733383062302465305037912912666797637939453125;0.35274989034390691333697986920014955103397369384765625;-0.475842857556607101710000051753013394773006439208984375;0.597827506479405190731313268770463764667510986328125;0.247242127543032041980808344305842183530330657958984375]
      mask Display: e = 0.06;c1 = [120 150 230]/255;c2 = ([120 150 230]+0)/383;c3 = ([120 150 230]+128)/383;patch([0 1 1 0],[0 0 1 1],c1);patch([0 1 1 1-e 1-e 0+e],[0 0 1 1-e 0+e 0+e],c2);patch([0 0 1 1-e 0+e 0+e],[0 1 1 1-e 1-e 0+e],c3);plot([0 1 1 0 0],[0 0 1 1 0]);disp('Weights');
  "IW{1,1}(55,:)'" : Constant  Value=[1.8098193413499281678724628363852389156818389892578125;-0.09592364790899783610900186658909660764038562774658203125;-1.1330799946994758453655549601535312831401824951171875;0.5919175716670486142589879818842746317386627197265625;-1.044925954678059820679436597856692969799041748046875;-0.3521206025328933453266699871164746582508087158203125;-0.231675457456909816844614624642417766153812408447265625;-0.55055218187395116302695896592922508716583251953125]
      mask Display: e = 0.06;c1 = [120 150 230]/255;c2 = ([120 150 230]+0)/383;c3 = ([120 150 230]+128)/383;patch([0 1 1 0],[0 0 1 1],c1);patch([0 1 1 1-e 1-e 0+e],[0 0 1 1-e 0+e 0+e],c2);patch([0 0 1 1-e 0+e 0+e],[0 1 1 1-e 1-e 0+e],c3);plot([0 1 1 0 0],[0 0 1 1 0]);disp('Weights');
  "IW{1,1}(56,:)'" : Constant  Value=[0.49524675244069238377875308287912048399448394775390625;-0.32085303463104819510220977463177405297756195068359375;1.5868530634614510521629426875733770430088043212890625;0.07934255612787487199621949685024446807801723480224609375;-0.049147746670952723035963316533525357954204082489013671875;-0.167621864207881554609258500931900925934314727783203125;-0.10239989093653291407637340171277173794806003570556640625;0.89053530073892372964650121502927504479885101318359375]
      mask Display: e = 0.06;c1 = [120 150 230]/255;c2 = ([120 150 230]+0)/383;c3 = ([120 150 230]+128)/383;patch([0 1 1 0],[0 0 1 1],c1);patch([0 1 1 1-e 1-e 0+e],[0 0 1 1-e 0+e 0+e],c2);patch([0 0 1 1-e 0+e 0+e],[0 1 1 1-e 1-e 0+e],c3);plot([0 1 1 0 0],[0 0 1 1 0]);disp('Weights');
  "IW{1,1}(57,:)'" : Constant  Value=[-0.004584091751976726754336244340493067284114658832550048828125;0.57095023784875997829857396936859004199504852294921875;0.99630031803517249411328293717815540730953216552734375;-0.448051294260545851511068349282140843570232391357421875;-0.1349218039294430848684669399517588317394256591796875;0.0024354417994565317855115704759327854844741523265838623046875;-1.35698026197675147841437137685716152191162109375;1.2156977434970961393645438874955289065837860107421875]
      mask Display: e = 0.06;c1 = [120 150 230]/255;c2 = ([120 150 230]+0)/383;c3 = ([120 150 230]+128)/383;patch([0 1 1 0],[0 0 1 1],c1);patch([0 1 1 1-e 1-e 0+e],[0 0 1 1-e 0+e 0+e],c2);patch([0 0 1 1-e 0+e 0+e],[0 1 1 1-e 1-e 0+e],c3);plot([0 1 1 0 0],[0 0 1 1 0]);disp('Weights');
  "IW{1,1}(58,:)'" : Constant  Value=[-0.43613854272731555905551203977665863931179046630859375;-0.259467967369604701755037012844695709645748138427734375;-0.2173661717909125268288761390067520551383495330810546875;1.3584206321968093078567108022980391979217529296875;-0.8707305475482562950872988949413411319255828857421875;1.0281351707122923233583833280135877430438995361328125;0.054981595812180726612350412096930085681378841400146484375;-1.2269974152258769084511413893778808414936065673828125]
      mask Display: e = 0.06;c1 = [120 150 230]/255;c2 = ([120 150 230]+0)/383;c3 = ([120 150 230]+128)/383;patch([0 1 1 0],[0 0 1 1],c1);patch([0 1 1 1-e 1-e 0+e],[0 0 1 1-e 0+e 0+e],c2);patch([0 0 1 1-e 0+e 0+e],[0 1 1 1-e 1-e 0+e],c3);plot([0 1 1 0 0],[0 0 1 1 0]);disp('Weights');
  "IW{1,1}(59,:)'" : Constant  Value=[0.57912934968435758609217600678675808012485504150390625;-0.019169885476493231379890858079306781291961669921875;1.048224020115640531258804912795312702655792236328125;-1.07616784288998434959694350254721939563751220703125;1.053626695484267461466743043274618685245513916015625;-0.638475744430138991702960993279702961444854736328125;1.3358629448222665292433930517290718853473663330078125;0.325749410027561914215965543917263858020305633544921875]
      mask Display: e = 0.06;c1 = [120 150 230]/255;c2 = ([120 150 230]+0)/383;c3 = ([120 150 230]+128)/383;patch([0 1 1 0],[0 0 1 1],c1);patch([0 1 1 1-e 1-e 0+e],[0 0 1 1-e 0+e 0+e],c2);patch([0 0 1 1-e 0+e 0+e],[0 1 1 1-e 1-e 0+e],c3);plot([0 1 1 0 0],[0 0 1 1 0]);disp('Weights');
  "IW{1,1}(6,:)'" : Constant  Value=[-0.5296965562707980357259884840459562838077545166015625;-0.38973649361983742078763270910712890326976776123046875;0.781382901275863961387813105829991400241851806640625;-1.8999187984653505001375606298097409307956695556640625;0.327049510341089810783188340792548842728137969970703125;0.97702923276992403867069469924899749457836151123046875;0.0751277132824597904114938273778534494340419769287109375;0.73976400624563887209461654492770321667194366455078125]
      mask Display: e = 0.06;c1 = [120 150 230]/255;c2 = ([120 150 230]+0)/383;c3 = ([120 150 230]+128)/383;patch([0 1 1 0],[0 0 1 1],c1);patch([0 1 1 1-e 1-e 0+e],[0 0 1 1-e 0+e 0+e],c2);patch([0 0 1 1-e 0+e 0+e],[0 1 1 1-e 1-e 0+e],c3);plot([0 1 1 0 0],[0 0 1 1 0]);disp('Weights');
  "IW{1,1}(60,:)'" : Constant  Value=[1.2508633191597102740644231744226999580860137939453125;-1.02487913267402586114940277184359729290008544921875;0.483219843313159092001995986720430664718151092529296875;-0.046964282878300685208916576129922759719192981719970703125;-0.930479706035839182476365749607793986797332763671875;-0.82052825178220090140968068226356990635395050048828125;-0.2486035869029936395957491868102806620299816131591796875;0.25107206350193089772204757537110708653926849365234375]
      mask Display: e = 0.06;c1 = [120 150 230]/255;c2 = ([120 150 230]+0)/383;c3 = ([120 150 230]+128)/383;patch([0 1 1 0],[0 0 1 1],c1);patch([0 1 1 1-e 1-e 0+e],[0 0 1 1-e 0+e 0+e],c2);patch([0 0 1 1-e 0+e 0+e],[0 1 1 1-e 1-e 0+e],c3);plot([0 1 1 0 0],[0 0 1 1 0]);disp('Weights');
  "IW{1,1}(7,:)'" : Constant  Value=[0.68032605516399258238635638917912729084491729736328125;-0.82607080608675909072502463459386490285396575927734375;0.57667091589975749688079531551920808851718902587890625;1.147983462953082511859292935696430504322052001953125;0.034658174975503421022526850947542698122560977935791015625;-0.26517017097192663310778470986406318843364715576171875;-1.271746072867304011566602639504708349704742431640625;-0.9235813199751683466587337534292601048946380615234375]
      mask Display: e = 0.06;c1 = [120 150 230]/255;c2 = ([120 150 230]+0)/383;c3 = ([120 150 230]+128)/383;patch([0 1 1 0],[0 0 1 1],c1);patch([0 1 1 1-e 1-e 0+e],[0 0 1 1-e 0+e 0+e],c2);patch([0 0 1 1-e 0+e 0+e],[0 1 1 1-e 1-e 0+e],c3);plot([0 1 1 0 0],[0 0 1 1 0]);disp('Weights');
  "IW{1,1}(8,:)'" : Constant  Value=[-0.2002158985673191671228465793319628573954105377197265625;1.2512917023421910034386428378638811409473419189453125;-0.3086854689243434535228516324423253536224365234375;1.4460723698274182691392297783750109374523162841796875;-0.810958505206266888620803001685999333858489990234375;-0.63250653250160071561225549885421060025691986083984375;0.420108068424603187107635449137887917459011077880859375;-0.08649545473259594163817354228740441612899303436279296875]
      mask Display: e = 0.06;c1 = [120 150 230]/255;c2 = ([120 150 230]+0)/383;c3 = ([120 150 230]+128)/383;patch([0 1 1 0],[0 0 1 1],c1);patch([0 1 1 1-e 1-e 0+e],[0 0 1 1-e 0+e 0+e],c2);patch([0 0 1 1-e 0+e 0+e],[0 1 1 1-e 1-e 0+e],c3);plot([0 1 1 0 0],[0 0 1 1 0]);disp('Weights');
  "IW{1,1}(9,:)'" : Constant  Value=[0.433515971015396128773744521822663955390453338623046875;0.7393100955140632368767228399519808590412139892578125;1.160413870956238380216518635279498994350433349609375;0.787274914069288289653059109696187078952789306640625;1.141160026323889464805461102514527738094329833984375;0.87966431079810314397349202408804558217525482177734375;-0.8784005081573618145540649493341334164142608642578125;0.42061155803675320807855086968629620969295501708984375]
      mask Display: e = 0.06;c1 = [120 150 230]/255;c2 = ([120 150 230]+0)/383;c3 = ([120 150 230]+128)/383;patch([0 1 1 0],[0 0 1 1],c1);patch([0 1 1 1-e 1-e 0+e],[0 0 1 1-e 0+e 0+e],c2);patch([0 0 1 1-e 0+e 0+e],[0 1 1 1-e 1-e 0+e],c3);plot([0 1 1 0 0],[0 0 1 1 0]);disp('Weights');
  Mux : Mux  Inputs=60
      mask Display: e = 0.06;c1 = [120 150 230]/255;c2 = ([120 150 230]+0)/383;c3 = ([120 150 230]+128)/383;patch([0 1 1 0],[0 0 1 1],c1);patch([0 1 1 1-e 1-e 0+e],[0 0 1 1-e 0+e 0+e],c2);patch([0 0 1 1-e 0+e 0+e],[0 1 1 1-e 1-e 0+e],c3);plot([0 1 1 0 0],[0 0 1 1 0]);disp('Mux');
  dotprod{1..60} (60 alike) : neural/Weight Functions/dotprod
  "iz{1,1}" : Outport
      mask Display: e = 0.06;c1 = [120 230 180]/255;c2 = ([120 230 180]+0)/(256+128);c3 = ([120 230 180]+128)/(256+128);patch([0 1 1 0],[0 0 1 1],c1);patch([0 1 1 1-e 1-e 0+e],[0 0 1 1-e 0+e 0+e],c2);patch([0 0 1 1-e 0+e 0+e],[0 1 1 1-e 1-e 0+e],c3);plot([0 1 1 0 0],[0 0 1 1 0]);
  wires:
  "IW{1,1}(1,:)'"/1 -> dotprod1/1
  "pd{1,1}"/1 -> dotprod1/2, dotprod2/2, dotprod3/2, dotprod4/2, dotprod5/2, dotprod6/2, dotprod7/2, dotprod8/2, dotprod9/2, dotprod10/2, dotprod11/2, dotprod12/2, dotprod13/2, dotprod14/2, dotprod15/2, dotprod16/2, dotprod17/2, dotprod18/2, dotprod19/2, dotprod20/2, dotprod21/2, dotprod22/2, dotprod23/2, dotprod24/2, dotprod25/2, dotprod26/2, dotprod27/2, dotprod28/2, dotprod29/2, dotprod30/2, dotprod31/2, dotprod32/2, dotprod33/2, dotprod34/2, dotprod35/2, dotprod36/2, dotprod37/2, dotprod38/2, dotprod39/2, dotprod40/2, dotprod41/2, dotprod42/2, dotprod43/2, dotprod44/2, dotprod45/2, dotprod46/2, dotprod47/2, dotprod48/2, dotprod49/2, dotprod50/2, dotprod51/2, dotprod52/2, dotprod53/2, dotprod54/2, dotprod55/2, dotprod56/2, dotprod57/2, dotprod58/2, dotprod59/2, dotprod60/2
  dotprod1/1 -> Mux/1
  "IW{1,1}(2,:)'"/1 -> dotprod2/1
  dotprod2/1 -> Mux/2
  "IW{1,1}(3,:)'"/1 -> dotprod3/1
  dotprod3/1 -> Mux/3
  "IW{1,1}(4,:)'"/1 -> dotprod4/1
  dotprod4/1 -> Mux/4
  "IW{1,1}(5,:)'"/1 -> dotprod5/1
  dotprod5/1 -> Mux/5
  "IW{1,1}(6,:)'"/1 -> dotprod6/1
  dotprod6/1 -> Mux/6
  "IW{1,1}(7,:)'"/1 -> dotprod7/1
  dotprod7/1 -> Mux/7
  "IW{1,1}(8,:)'"/1 -> dotprod8/1
  dotprod8/1 -> Mux/8
  "IW{1,1}(9,:)'"/1 -> dotprod9/1
  dotprod9/1 -> Mux/9
  "IW{1,1}(10,:)'"/1 -> dotprod10/1
  dotprod10/1 -> Mux/10
  "IW{1,1}(11,:)'"/1 -> dotprod11/1
  dotprod11/1 -> Mux/11
  "IW{1,1}(12,:)'"/1 -> dotprod12/1
  dotprod12/1 -> Mux/12
  "IW{1,1}(13,:)'"/1 -> dotprod13/1
  dotprod13/1 -> Mux/13
  "IW{1,1}(14,:)'"/1 -> dotprod14/1
  dotprod14/1 -> Mux/14
  "IW{1,1}(15,:)'"/1 -> dotprod15/1
  dotprod15/1 -> Mux/15
  "IW{1,1}(16,:)'"/1 -> dotprod16/1
  dotprod16/1 -> Mux/16
  "IW{1,1}(17,:)'"/1 -> dotprod17/1
  dotprod17/1 -> Mux/17
  "IW{1,1}(18,:)'"/1 -> dotprod18/1
  dotprod18/1 -> Mux/18
  "IW{1,1}(19,:)'"/1 -> dotprod19/1
  dotprod19/1 -> Mux/19
  "IW{1,1}(20,:)'"/1 -> dotprod20/1
  dotprod20/1 -> Mux/20
  "IW{1,1}(21,:)'"/1 -> dotprod21/1
  dotprod21/1 -> Mux/21
  "IW{1,1}(22,:)'"/1 -> dotprod22/1
  dotprod22/1 -> Mux/22
  "IW{1,1}(23,:)'"/1 -> dotprod23/1
  dotprod23/1 -> Mux/23
  "IW{1,1}(24,:)'"/1 -> dotprod24/1
  dotprod24/1 -> Mux/24
  "IW{1,1}(25,:)'"/1 -> dotprod25/1
  dotprod25/1 -> Mux/25
  "IW{1,1}(26,:)'"/1 -> dotprod26/1
  dotprod26/1 -> Mux/26
  "IW{1,1}(27,:)'"/1 -> dotprod27/1
  dotprod27/1 -> Mux/27
  "IW{1,1}(28,:)'"/1 -> dotprod28/1
  dotprod28/1 -> Mux/28
  "IW{1,1}(29,:)'"/1 -> dotprod29/1
  dotprod29/1 -> Mux/29
  "IW{1,1}(30,:)'"/1 -> dotprod30/1
  dotprod30/1 -> Mux/30
  "IW{1,1}(31,:)'"/1 -> dotprod31/1
  dotprod31/1 -> Mux/31
  "IW{1,1}(32,:)'"/1 -> dotprod32/1
  dotprod32/1 -> Mux/32
  "IW{1,1}(33,:)'"/1 -> dotprod33/1
  dotprod33/1 -> Mux/33
  "IW{1,1}(34,:)'"/1 -> dotprod34/1
  dotprod34/1 -> Mux/34
  "IW{1,1}(35,:)'"/1 -> dotprod35/1
  dotprod35/1 -> Mux/35
  "IW{1,1}(36,:)'"/1 -> dotprod36/1
  dotprod36/1 -> Mux/36
  "IW{1,1}(37,:)'"/1 -> dotprod37/1
  dotprod37/1 -> Mux/37
  "IW{1,1}(38,:)'"/1 -> dotprod38/1
  dotprod38/1 -> Mux/38
  "IW{1,1}(39,:)'"/1 -> dotprod39/1
  dotprod39/1 -> Mux/39
  "IW{1,1}(40,:)'"/1 -> dotprod40/1
  dotprod40/1 -> Mux/40
  "IW{1,1}(41,:)'"/1 -> dotprod41/1
  dotprod41/1 -> Mux/41
  "IW{1,1}(42,:)'"/1 -> dotprod42/1
  dotprod42/1 -> Mux/42
  "IW{1,1}(43,:)'"/1 -> dotprod43/1
  dotprod43/1 -> Mux/43
  "IW{1,1}(44,:)'"/1 -> dotprod44/1
  dotprod44/1 -> Mux/44
  "IW{1,1}(45,:)'"/1 -> dotprod45/1
  dotprod45/1 -> Mux/45
  "IW{1,1}(46,:)'"/1 -> dotprod46/1
  dotprod46/1 -> Mux/46
  "IW{1,1}(47,:)'"/1 -> dotprod47/1
  dotprod47/1 -> Mux/47
  "IW{1,1}(48,:)'"/1 -> dotprod48/1
  dotprod48/1 -> Mux/48
  "IW{1,1}(49,:)'"/1 -> dotprod49/1
  dotprod49/1 -> Mux/49
  "IW{1,1}(50,:)'"/1 -> dotprod50/1
  dotprod50/1 -> Mux/50
  "IW{1,1}(51,:)'"/1 -> dotprod51/1
  dotprod51/1 -> Mux/51
  "IW{1,1}(52,:)'"/1 -> dotprod52/1
  dotprod52/1 -> Mux/52
  "IW{1,1}(53,:)'"/1 -> dotprod53/1
  dotprod53/1 -> Mux/53
  "IW{1,1}(54,:)'"/1 -> dotprod54/1
  dotprod54/1 -> Mux/54
  "IW{1,1}(55,:)'"/1 -> dotprod55/1
  dotprod55/1 -> Mux/55
  "IW{1,1}(56,:)'"/1 -> dotprod56/1
  dotprod56/1 -> Mux/56
  "IW{1,1}(57,:)'"/1 -> dotprod57/1
  dotprod57/1 -> Mux/57
  "IW{1,1}(58,:)'"/1 -> dotprod58/1
  dotprod58/1 -> Mux/58
  "IW{1,1}(59,:)'"/1 -> dotprod59/1
  dotprod59/1 -> Mux/59
  "IW{1,1}(60,:)'"/1 -> dotprod60/1
  dotprod60/1 -> Mux/60
  Mux/1 -> "iz{1,1}"/1
